simulink model "sldemo_mdlref_dsm"  (Simulink 7.6)
settings: Solver=FixedStepDiscrete  StartTime=0.0  StopTime=10.0  FixedStep=0.1  RelTol=1e-3
PreLoadFcn:
  | load sldemo_mdlref_dsm_data.mat
Description:
  | Model Reference and Global Data Stores
  | 
  | This demonstration explains how to define and use global data stores to
  | share global data among reference models.
settings Model: Creator=The MathWorks Inc.  ExtModeAutoUpdateStatusClock=off
settings OptimizationCC: InlineParams=on  InitFltsAndDblsToZero=on
settings DebuggingCC: SaveWithParameterizedLinksMsg=none  MultiTaskCondExecSysMsg=none  SigSpecEnsureSampleTimeMsg=none  BusObjectLabelMismatch=error  RootOutportRequireBusObject=error  StrictBusMsg=ErrorOnBusTreatedAsVector
settings ModelReferenceCC: UpdateModelReferenceTargets=IfOutOfDate
settings RTWCC: ProcessScript=grt_make_rtw_hook  IncludeERTFirstTime=on
settings CodeAppCC: MaxIdLength=100
settings GRTTargetCC: TargetFcnLib=ansi_tfl_tmw.mat

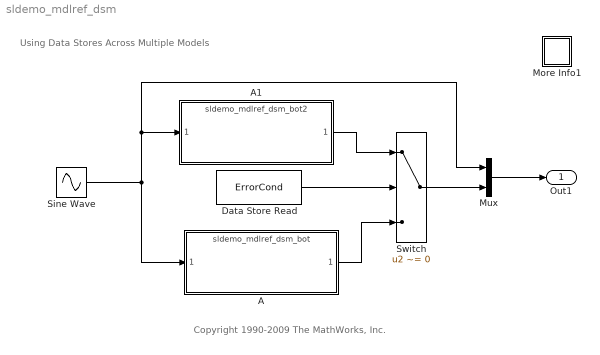
== system sldemo_mdlref_dsm ==
  note: Copyright 1990-2009 The MathWorks, Inc.
  note: Using Data Stores Across Multiple Models
  A : ModelReference  ModelNameDialog=sldemo_mdlref_dsm_bot  SimulationMode=Normal  ModelReferenceVersion=1.53  CopyOfModelName=sldemo_mdlref_dsm_bot
  A1 : ModelReference  ModelNameDialog=sldemo_mdlref_dsm_bot2  SimulationMode=Normal  ModelReferenceVersion=1.34  CopyOfModelName=sldemo_mdlref_dsm_bot2
  Data Store Read : DataStoreRead  DataStoreName=ErrorCond  SampleTime=0.1
  More Info1 : Subsystem
      settings: OpenFcn=showdemo(bdroot(gcb))
      mask Display: disp('?')
  Mux : Mux  Inputs=2
  Sine Wave : Sin  SampleTime=0.1
  Switch : Switch  Criteria=u2 ~= 0
  Out1 : Outport
  wires:
  Sine Wave/1 -> Mux/1, A1/1, A/1
  Data Store Read/1 -> Switch/2
  Switch/1 -> Mux/2
  Mux/1 -> Out1/1
  A1/1 -> Switch/1
  A/1 -> Switch/3

== system sldemo_mdlref_dsm/More Info1 ==
